simulink model "BCG_model"  (R2017a)
settings: Solver=FixedStepDiscrete  StartTime=0.0  StopTime=inf  RelTol=1e-3
undefined symbols (not defined in the file): Saa, Sab, Sda, Sic, vaa, vab, vda, vic
settings Model: Creator=Samuel  LastModifiedBy=Samuel
settings SolverCC: AutoInsertRateTranBlk=on
settings DataIOCC: LimitDataPoints=on  SaveOutput=off  SignalLogging=off  SaveTime=off
settings OptimizationCC: LifeSpan=inf
settings DebuggingCC: AlgebraicLoopMsg=error  SingleTaskRateTransMsg=error  AllowSymbolicDim=off  SFUnexpectedBacktrackingDiag=warning  SFNoUnconditionalDefaultTransitionDiag=warning  SFExecutionAtInitializationDiag=none
settings GRTTargetCC: TargetLangStandard=C89/C90 (ANSI)  GeneratePreprocessorConditionals=Disable all

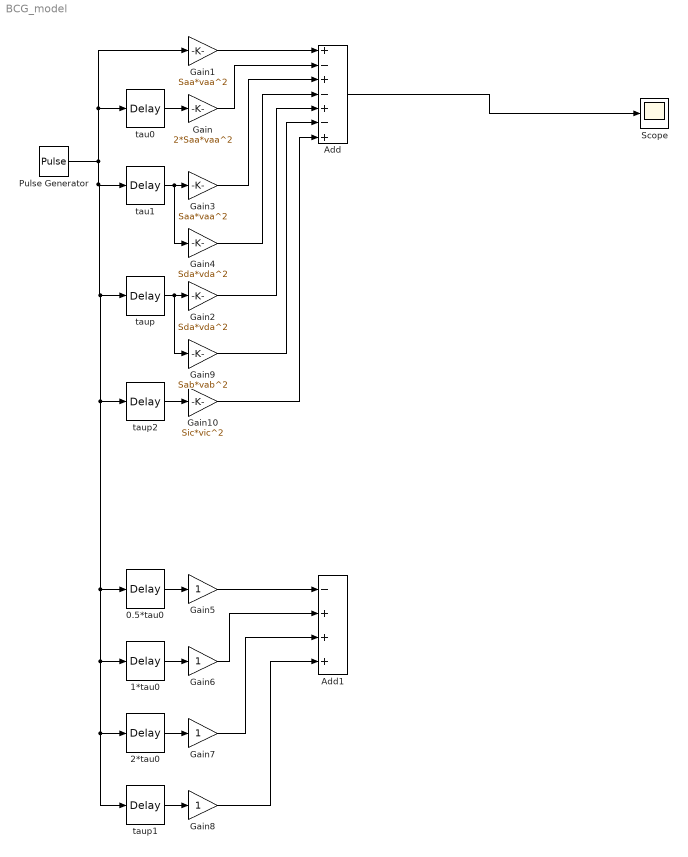
== system BCG_model ==
  0.5*tau0 : TransportDelay  DelayTime=0.05
  1*tau0 : TransportDelay  DelayTime=0.1
  2*tau0 : TransportDelay  DelayTime=0.2
  Add : Sum  Inputs=+-+-+-+
  Add1 : Sum  Inputs=-+++
  Gain : Gain  Gain=2*Saa*vaa^2
  Gain1 : Gain  Gain=Saa*vaa^2
  Gain10 : Gain  Gain=Sic*vic^2
  Gain2 : Gain  Gain=Sda*vda^2
  Gain3 : Gain  Gain=Saa*vaa^2
  Gain4 : Gain  Gain=Sda*vda^2
  Gain{5..8} (4 alike) : Gain
  Gain9 : Gain  Gain=Sab*vab^2
  Pulse Generator : DiscretePulseGenerator  PulseType=Time based  Period=1  PulseWidth=5
  Scope : Scope
  tau0 : TransportDelay  DelayTime=0.1
  tau1 : TransportDelay  DelayTime=0.6
  taup : TransportDelay  DelayTime=0.8
  taup1 : TransportDelay  DelayTime=2.8
  taup2 : TransportDelay  DelayTime=0.9
  wires:
  Pulse Generator/1 -> taup2/1, taup1/1, 2*tau0/1, 1*tau0/1, 0.5*tau0/1, taup/1, tau1/1, tau0/1, Gain1/1
  Gain1/1 -> Add/1
  Gain/1 -> Add/2
  Gain3/1 -> Add/3
  Gain4/1 -> Add/4
  tau1/1 -> Gain4/1, Gain3/1
  tau0/1 -> Gain/1
  taup/1 -> Gain9/1, Gain2/1
  Gain2/1 -> Add/5
  0.5*tau0/1 -> Gain5/1
  1*tau0/1 -> Gain6/1
  2*tau0/1 -> Gain7/1
  taup1/1 -> Gain8/1
  Gain5/1 -> Add1/1
  Gain6/1 -> Add1/2
  Gain7/1 -> Add1/3
  Gain8/1 -> Add1/4
  Add/1 -> Scope/1
  taup2/1 -> Gain10/1
  Gain9/1 -> Add/6
  Gain10/1 -> Add/7
